simulink subsystem "PvtSubSys_PLAN_AP"  (R2020b)
settings: Solver=VariableStepAuto  StartTime=0.0  StopTime=10.0  RelTol=1e-3
undefined symbols (not defined in the file or in its folder): C_LongCtrl_0_Single, C_LongCtrl_0_Uint8, C_LongCtrl_Mph2Kph, magnitude, P_LongCtrl_accelTargAbsThrd, P_LongCtrl_AddVelAccelChange, P_LongCtrl_AddVelAccelThrd, P_LongCtrl_AddVelDistDesThrd, P_LongCtrl_AddVelEnable, P_LongCtrl_AddVelRefMsThrd, P_LongCtrl_ALaLowerChar, P_LongCtrl_ALaUpperCharEco, P_LongCtrl_ALaUpperCharNormal, P_LongCtrl_ALaUpperCharSport, P_LongCtrl_ALCAccLimitByDangerXAxis, P_LongCtrl_ALCAccLimitByDangerYAxis, P_LongCtrl_ALvAcceleLowerChar, P_LongCtrl_ALvAcceleUpperCharEco, P_LongCtrl_ALvAcceleUpperCharNormal, P_LongCtrl_ALvAcceleUpperCharSport, P_LongCtrl_CCaccelCCNeg2PosJerk, P_LongCtrl_CCaccelCCPosJerk, P_LongCtrl_CCaccelLowerIsLaneChange, P_LongCtrl_CCaccelMaxLCActive, P_LongCtrl_CCaccelMinECOAL, P_LongCtrl_CCaccelMinFastDecel, P_LongCtrl_CCaccelMinNoFastDecel, P_LongCtrl_CCaccelMinNormAL, P_LongCtrl_CCaccelMinSportAL, P_LongCtrl_CCaccelUpperCC, P_LongCtrl_CCaccelUpperCCSafeStop, P_LongCtrl_CCaMinNegAcceleLowerBand, P_LongCtrl_CCaMinNegAcceleUpperBand, P_LongCtrl_CCaMinPosAcceleLowerBand, P_LongCtrl_CCaMinPosAcceleUpperBand, P_LongCtrl_CCbECO, P_LongCtrl_CCbNorm, P_LongCtrl_CCbSport, P_LongCtrl_CCcoefESPSpd2IPSpd1, P_LongCtrl_CCcoefESPSpd2IPSpd2, P_LongCtrl_CCdecelCCJerk, P_LongCtrl_CCdecelCCJerkNegVLCInternalAcc, P_LongCtrl_CCfacNegAcceleLowerBand, P_LongCtrl_CCfacNegAcceleUpperBand, P_LongCtrl_CCfacPosAcceleLowerBand, P_LongCtrl_CCfacPosAcceleUpperBand, P_LongCtrl_CCkECO, P_LongCtrl_CCkNorm, P_LongCtrl_CCkSport, P_LongCtrl_CCLCIncSetSpdAdd, P_LongCtrl_CCLCIncSetSpdAddCntStartValue, P_LongCtrl_CCResumeDelayDeltaVel, P_LongCtrl_CCtAcceleTimeNeg, P_LongCtrl_CCtAcceleTimeNegCorrXAxis, P_LongCtrl_CCtAcceleTimeNegCorrYAxis, P_LongCtrl_CCtAcceleTimePos, P_LongCtrl_CCtAcceleTimePosCorrXAxis, P_LongCtrl_CCtAcceleTimePosCorrYAxis, P_LongCtrl_CCtStepVelPlan, P_LongCtrl_CCtTotVelPlan ... (+150)
libraries: simulink x62, TrueDurationTime x1
(part 1 of 7)
settings Model: Creator=GW00202955  LastModifiedBy=GW00235400

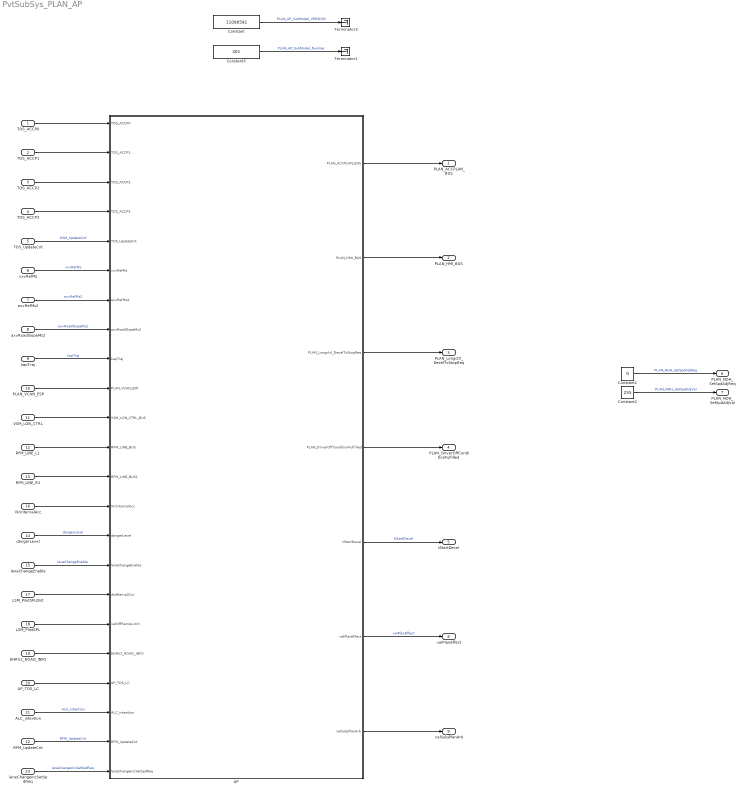
== system PvtSubSys_PLAN_AP ==
  TOS_ACCP0 : Inport  Description=|  OutDataTypeStr=Bus: TOS_ACCP0_BUS  PortDimensions=1  BusOutputAsStruct=on
      | IDP0     P0目标ID，确定目标是否切换
      | vxRelP0         P0目标相对速度，计算跟车加速度
      | axAbsGroundP0   P0目标绝对加速度，计算跟车加速度
      | rangeP0         P0目标相对距离，计算跟车加速度及P0动态距离
      | targetExistP0   P0目标是否存在，计算跟车加速度
      | ObjTypeP0       P0类型
  TOS_ACCP1 : Inport  Port=2  OutDataTypeStr=Bus: TOS_ACCP1_BUS  PortDimensions=1  BusOutputAsStruct=on
  TOS_ACCP2 : Inport  Description=|  Port=3  OutDataTypeStr=Bus: TOS_ACCP2_BUS  PortDimensions=1  BusOutputAsStruct=on
      | IDP2                 P2目标ID，确定目标是否切换
      | axAbsGroundP2        P2目标绝对加速度，计算P0目标绝对加速度滤波
      | rangeP2              P2目标相对距离，计算P2目标动态距离
      | targetExistP2        P2目标是否存在，计算P2目标动态距离
  TOS_ACCP3 : Inport  Description=|  Port=4  OutDataTypeStr=Bus: TOS_ACCP3_BUS  PortDimensions=1  BusOutputAsStruct=on
      | IDP3                 P3目标ID，确定目标是否切换
      | axAbsGroundP3        P3目标绝对加速度，计算P0目标绝对加速度滤波
      | rangeP3              P3目标相对距离，计算P2目标动态距离
      | targetExistP3        P3目标是否存在，计算P2目标动态距离
  TOS_UpdateCnt : Inport  Description=|目标是否更新  Port=5  OutDataTypeStr=uint32  PortDimensions=1  BusOutputAsStruct=on
  vxvRefMs : Inport  Description=m/s |车速  Port=6  OutDataTypeStr=single  PortDimensions=1  BusOutputAsStruct=on
  axvRefMs2 : Inport  Description=m/s^2 |自车参考加速度（未考虑CAN）  Port=7  OutDataTypeStr=single  PortDimensions=1  BusOutputAsStruct=on
  axvRoadSlopeMs2 : Inport  Description="m/s^2  |坡道加速度"  Port=8  OutDataTypeStr=single  PortDimensions=1  BusOutputAsStruct=on
  kapTraj : Inport  Description=1/m |方向盘转角计算弯道曲率，计算弯道工况加速度  Port=9  OutDataTypeStr=single  PortDimensions=1  BusOutputAsStruct=on
  PLAN_VCAN_ESP : Inport  Description=|  Port=10  OutDataTypeStr=Bus: VCAN_ESP_MSG_BUS  PortDimensions=1  BusOutputAsStruct=on
      | VehSpd   车速，用于计算仪表显示车速
      | DrivingModDis   驾驶模式
  VSM_LON_CTRL : Inport  Description=|  Port=11  OutDataTypeStr=Bus: VSM_LON_CTRL_BUS  PortDimensions=1  BusOutputAsStruct=on
      | ACCSts                 ACC状态
      | ACC_SpdSetValueKmh     驾驶员设定巡航速度
      | ACC_TimeGapSet         驾驶员设定车间时距
      | vSetBelowMin           驾驶员期望设定速度低于最小设定速度
      | HWAAccControlSts       HWA状态，用来判断换道进行中、safestop、HWA慢退
  RFM_LINE_L1 : Inport  Description=|  Port=12  OutDataTypeStr=Bus: RFM_LINE_BUS  PortDimensions=1  BusOutputAsStruct=on
      | dC0V          左侧车道线三次多项式常数项系数
      | dC1V          左侧车道线三次多项式一次项系数     
      | dC2V          左侧车道线三次多项式二次项系数  
      | dC3V          左侧车道线三次多项式三次项系数  
      | dDisFront     车辆坐标系X方向车道线置信距离
      | bIsLineExist  车道线存在
  RFM_LINE_R1 : Inport  Description=|  Port=13  OutDataTypeStr=Bus: RFM_LINE_BUS  PortDimensions=1  BusOutputAsStruct=on
      | dC0V          右侧车道线三次多项式常数项系数
      | dC1V          右侧车道线三次多项式一次项系数     
      | dC2V          右侧车道线三次多项式二次项系数  
      | dC3V          右侧车道线三次多项式三次项系数  
      | dDisFront     车辆坐标系X方向车道线置信距离
      | bIsLineExist  车道线存在
  dangerLevel : Inport  Description=|换道危险程度，抑制换道减速度  Port=14  OutDataTypeStr=single  PortDimensions=1
  laneChangeEnable : Inport  Description=|换道条件满足，用作换道减速度抑制开启条件  Port=15  OutDataTypeStr=boolean  PortDimensions=1
  VlcInternalAcc : Inport  Description=m/s^2 |VLC执行加速度，用作当前加速度判断  Port=16  OutDataTypeStr=single  PortDimensions=1
  LSM_PilotSPLDist : Inport  Description=m |到匝道距离  Port=17  OutDataTypeStr=uint16  PortDimensions=1
  LSM_PilotSPL : Inport  Description=km/h |匝道限速  Port=18  OutDataTypeStr=uint8  PortDimensions=1
  EHRV2_ROAD_INFO : Inport  Description=|  Port=19  OutDataTypeStr=Bus: EHRV2_ROAD_INFO_BUS
      | i_road_curvature                    当前车辆位置处曲率(左正右负)
      | i_road_curvature_far                当前车辆位置前方Xm内最大曲率(左正右负)
      | i_road_curvature_far_distance       当前车辆位置与前方Xm内最大曲率点相对距离
      | i_road_curvature_value_matrix       车辆所在车道道路记录点的曲率组成的矩阵
      | i_road_curvature_distance_matrix    车辆坐标系下道路记录点的x坐标组成的矩阵
      | i_road_curvature_matrix_size        车辆所在车道道路记录点的个数
  AP_TOS_LC : Inport  Description=|  Port=20  OutDataTypeStr=Bus: TOS_LC_BUS
      | Object_ID             融合追踪处理后，目标的ID
      | Object_Type           目标的类型（行人、小汽车、卡车...）
      | Object_Length         目标的长度
      | Object_Width          目标的宽度
      | Object_Hight          目标的高度
      | Object_DX             车体坐标系下，自车和目标纵向相对距离
      | Object_DY             车体坐标系下，自车和目标横向相对距离
      | Object_VX             目标的纵向的速度
      | Object_VY             目标的横向的速度
      | Object_HeadingAngle   车体系下, 目标航向角
      | Object_Fus_Type       目标是否是融合,传感器类型
      | Object_ExistProb      目标存在的可能性
      | Object_ObstacleProb   目标成为障碍物的概率值
      | Object_Age            目标存在生命周期
      | Object_AX             目标的纵向的加速度
  ALC_intention : Inport  Description="|  换到意图 -1右换道，0不换"  Port=21  OutDataTypeStr=int8  PortDimensions=1
  RFM_UpdateCnt : Inport  Description=|RFM更新周期  Port=22  OutDataTypeStr=uint32  PortDimensions=1
  laneChangeIncSetSpdReq : Inport  Description=|换道加速开启条件  Port=23  OutDataTypeStr=uint8  PortDimensions=1
  AP : Subsystem  Description=Acceleration Plan
  Constant : Constant  Value=11090591  OutDataTypeStr=uint32
  Constant1 : Constant  Value=0  OutDataTypeStr=boolean
  Constant2 : Constant  Value=255  OutDataTypeStr=uint8
  Constant3 : Constant  Value=301  OutDataTypeStr=uint32
  Terminator1 : Terminator
  Terminator3 : Terminator
  PLAN_ACCPLAN_BUS : Outport  Description=|  OutDataTypeStr=Bus: PLAN_ACCPLAN_BUS
      | ACC_axvCvAim                      期望加速度
      | ACC_axv_ComfortBandLowerValue     期望加速度下限
      | ACC_axv_ComfortBandUpperValue     期望加速度上限
      | ACC_DecelerateJerk                加速度变化率下限
      | ACC_AccelerateJerk                加速度变化率上限         
      | ACC_BrakePrefer                   制动优先
  PLAN_HMI_BUS : Outport  Description=|  Port=2  OutDataTypeStr=Bus: PLAN_HMI_BUS
      | tor                       驾驶员接管请求
      | ACC_TgtObjBarDisp         P0动态距离
      | ACC_LeTgtObjBarDisp       P2动态距离
      | ACC_RiTgtObjBarDisp       P3动态距离
      | IntelligentCurveActive    智能过弯激活状态
  PLAN_Longctrl_DecelToStopReq : Outport  Description=|制动到停状态  Port=3  OutDataTypeStr=boolean  PortDimensions=1
  PLAN_DriverOffConditionFulfilled : Outport  Description=|起步条件满足  Port=4  OutDataTypeStr=boolean  PortDimensions=1
  tStartDecel : Outport  Port=5
  PLAN_NOH_SetSpdAdjReq : Outport  Port=6  OutDataTypeStr=boolean
  PLAN_NOH_SetSpdAdjVal : Outport  Port=7  OutDataTypeStr=uint8
  velPlanEffect : Outport  Port=8
  velSubjPlanArb : Outport  Port=9
  wires:
  VSM_LON_CTRL/1 -> AP/11(VSM_LON_CTRL_BUS)
  Constant3/1 -> Terminator1/1  "PLAN_AP_SubModel_Number"
  laneChangeIncSetSpdReq/1 -> AP/23(laneChangeIncSetSpdReq)  "laneChangeIncSetSpdReq"
  axvRoadSlopeMs2/1 -> AP/8(axvRoadSlopeMs2)  "axvRoadSlopeMs2"
  LSM_PilotSPL/1 -> AP/18(velOffRampLimit)
  dangerLevel/1 -> AP/15(dangerLevel)  "dangerLevel"
  AP/2(PLAN_HMI_BUS) -> PLAN_HMI_BUS/1
  TOS_UpdateCnt/1 -> AP/5(TOS_UpdateCnt)  "OSM_UpdateCnt"
  LSM_PilotSPLDist/1 -> AP/17(distRamp2Cur)
  AP/1(PLAN_ACCPLAN_BUS) -> PLAN_ACCPLAN_BUS/1
  Constant/1 -> Terminator3/1  "PLAN_AP_SubModel_VERSION"
  vxvRefMs/1 -> AP/6(vxvRefMs)  "vxvRefMs"
  kapTraj/1 -> AP/9(kapTraj)  "kapTraj"
  TOS_ACCP1/1 -> AP/2(TOS_ACCP1)
  RFM_LINE_R1/1 -> AP/13(RFM_LINE_BUS1)
  TOS_ACCP2/1 -> AP/3(TOS_ACCP2)
  TOS_ACCP0/1 -> AP/1(TOS_ACCP0)
  AP/3(PLAN_Longctrl_DecelToStopReq) -> PLAN_Longctrl_DecelToStopReq/1
  PLAN_VCAN_ESP/1 -> AP/10(PLAN_VCAN_ESP)
  AP/5(tStartDecel) -> tStartDecel/1  "tStartDecel"
  Constant1/1 -> PLAN_NOH_SetSpdAdjReq/1  "PLAN_NOH_SetSpdAdjReq"
  RFM_UpdateCnt/1 -> AP/22(RFM_UpdateCnt)  "RFM_UpdateCnt"
  TOS_ACCP3/1 -> AP/4(TOS_ACCP3)
  VlcInternalAcc/1 -> AP/14(VlcInternalAcc)
  ALC_intention/1 -> AP/21(ALC_intention)  "ALC_intention"
  RFM_LINE_L1/1 -> AP/12(RFM_LINE_BUS)
  Constant2/1 -> PLAN_NOH_SetSpdAdjVal/1  "PLAN_NOH_SetSpdAdjVal"
  laneChangeEnable/1 -> AP/16(laneChangeEnable)  "laneChangeEnable"
  axvRefMs2/1 -> AP/7(axvRefMs2)  "axvRefMs2"
  AP/7(velSubjPlanArb) -> velSubjPlanArb/1
  AP/4(PLAN_DriverOffConditionFulfilled) -> PLAN_DriverOffConditionFulfilled/1
  EHRV2_ROAD_INFO/1 -> AP/19(EHRV2_ROAD_INFO)
  AP/6(velPlanEffect) -> velPlanEffect/1  "velPlanEffect"
  AP_TOS_LC/1 -> AP/20(AP_TOS_LC)

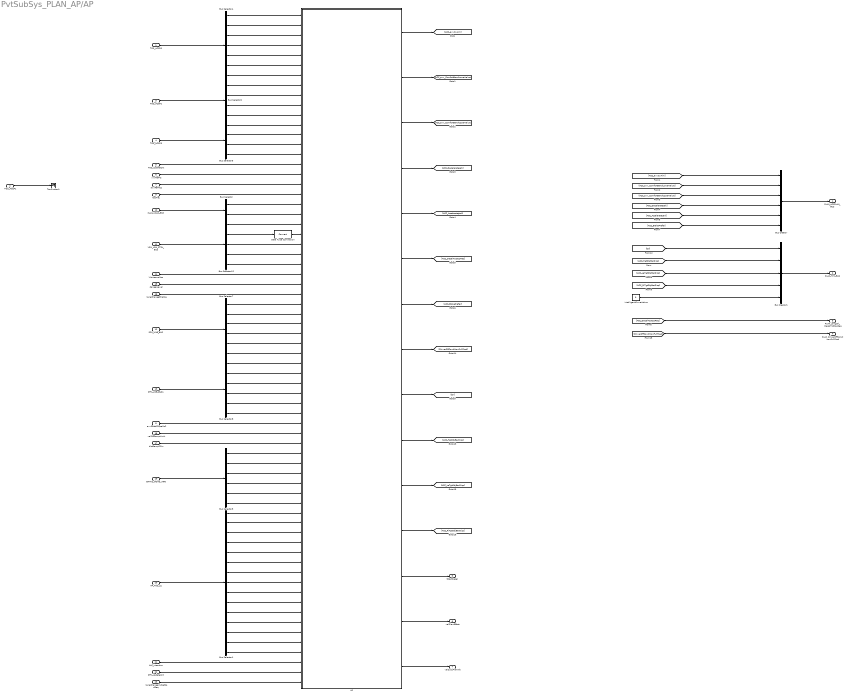
== system PvtSubSys_PLAN_AP/AP ==
  TOS_ACCP0 : Inport  OutDataTypeStr=Bus: TOS_ACCP0_BUS  LockScale=on
  TOS_ACCP1 : Inport  Port=2  OutDataTypeStr=Bus: TOS_ACCP1_BUS
  TOS_ACCP2 : Inport  Port=3  OutDataTypeStr=Bus: TOS_ACCP2_BUS
  TOS_ACCP3 : Inport  Port=4  OutDataTypeStr=Bus: TOS_ACCP3_BUS
  TOS_UpdateCnt : Inport  Port=5
  vxvRefMs : Inport  Port=6
  axvRefMs2 : Inport  Port=7
  axvRoadSlopeMs2 : Inport  Port=8
  kapTraj : Inport  Port=9
  PLAN_VCAN_ESP : Inport  Port=10  OutDataTypeStr=Bus: VCAN_ESP_MSG_BUS
  VSM_LON_CTRL_BUS : Inport  Port=11  OutDataTypeStr=Bus: VSM_LON_CTRL_BUS
  RFM_LINE_BUS : Inport  Port=12  OutDataTypeStr=Bus: RFM_LINE_BUS
  RFM_LINE_BUS1 : Inport  Port=13  OutDataTypeStr=Bus: RFM_LINE_BUS
  VlcInternalAcc : Inport  Port=14
  dangerLevel : Inport  Port=15
  laneChangeEnable : Inport  Port=16
  distRamp2Cur : Inport  Port=17  OutDataTypeStr=uint16
  velOffRampLimit : Inport  Port=18  OutDataTypeStr=uint8
  EHRV2_ROAD_INFO : Inport  Port=19  OutDataTypeStr=Bus: EHRV2_ROAD_INFO_BUS
  AP_TOS_LC : Inport  Port=20  OutDataTypeStr=Bus: TOS_LC_BUS
  ALC_intention : Inport  Port=21
  RFM_UpdateCnt : Inport  Port=22  OutDataTypeStr=uint32
  laneChangeIncSetSpdReq : Inport  Port=23  OutDataTypeStr=uint8
  AP : Subsystem  Description=Acceleration Plan  TreatAsAtomicUnit=on
  Bus Creator : BusCreator  Inputs=6  OutDataTypeStr=Bus: PLAN_ACCPLAN_BUS  NonVirtualBus=on
      settings: InheritFromInputs=off
  Bus Creator1 : BusCreator  Inputs=5  OutDataTypeStr=Bus: PLAN_HMI_BUS  NonVirtualBus=on
      settings: InheritFromInputs=off
  Bus Selector : BusSelector  OutputSignals=VehSpd,DrivingModDis
  Bus Selector1 : BusSelector  OutputSignals=Object_ID,Object_Type,Object_Length,Object_Width,Object_Hight,Object_DX,Object_DY,Object_VX,Object_VY,Object_HeadingAngle,Object_Fus_Type,Object_ExistProb,Object_ObstacleProb,Object_Age,Object_AX
  Bus Selector12 : BusSelector  OutputSignals=ACCSts,ACC_SpdSetValueKmh,ACC_TimeGapSet,vSetBelowMin,HWAAccControlSts
  Bus Selector2 : BusSelector  OutputSignals=IDP2,axAbsGroundP2,rangeP2,targetExistP2
  Bus Selector3 : BusSelector  OutputSignals=i_road_curvature,i_road_curvature_far,i_road_curvature_far_distance,i_road_curvature_value_matrix,i_road_curvature_distance_matrix,i_road_curvature_matrix_size
  Bus Selector4 : BusSelector  OutputSignals=IDP0,vxRelP0,axAbsGroundP0,rangeP0,targetExistP0,ObjTypeP0,ObjMovingStateP0
  Bus Selector5 : BusSelector  OutputSignals=IDP3,axAbsGroundP3,rangeP3,targetExistP3
  Bus Selector7 : BusSelector  OutputSignals=dC0V,dC1V,dC2V,dC3V,dDisFront,bIsLineExist
  Bus Selector8 : BusSelector  OutputSignals=dC0V,dC1V,dC2V,dC3V,dDisFront,bIsLineExist
  Data Type Conversion : DataTypeConversion
  IntelligentCurveActive : Constant  Value=0  OutDataTypeStr=boolean
  Terminator1 : Terminator
  PLAN_ACCPLAN_BUS : Outport  OutDataTypeStr=Bus: PLAN_ACCPLAN_BUS
  PLAN_HMI_BUS : Outport  Port=2  OutDataTypeStr=Bus: PLAN_HMI_BUS
  PLAN_Longctrl_DecelToStopReq : Outport  Port=3  OutDataTypeStr=boolean
  PLAN_DriverOffConditionFulfilled : Outport  Port=4  OutDataTypeStr=boolean
  tStartDecel : Outport  Port=5  OutDataTypeStr=single
  velPlanEffect : Outport  Port=6  OutDataTypeStr=uint8
  velSubjPlanArb : Outport  Port=7  OutDataTypeStr=single
  wires:
  Bus Selector4/7 -> AP/7(ObjMovingStateP0)  "<ObjMovingStateP0>"
  Bus Selector4/6 -> AP/6(ObjTypeP0)  "<ObjTypeP0>"
  RFM_UpdateCnt/1 -> AP/67(RFM_UpdateCnt)  "RFM_UpdateCnt"
  Bus Selector1/4 -> AP/54(Object_Width)  "<Object_Width>"
  Bus Selector1/9 -> AP/59(Object_VY)  "<Object_VY>"
  Bus Selector1/11 -> AP/61(Object_Fus_Type)  "<Object_Fus_Type>"
  Bus Selector1/8 -> AP/58(Object_VX)  "<Object_VX>"
  Bus Selector3/4 -> AP/48(i_road_curvature_value_matrix)  "<i_road_curvature_value_matrix>"
  Bus Selector1/13 -> AP/63(Object_ObstacleProb)  "<Object_ObstacleProb>"
  Bus Selector1/12 -> AP/62(Object_ExistProb)  "<Object_ExistProb>"
  Bus Selector1/15 -> AP/65(Object_AX)  "<Object_AX>"
  Bus Selector1/14 -> AP/64(Object_Age)  "<Object_Age>"
  Bus Selector3/1 -> AP/45(i_road_curvature)  "<i_road_curvature>"
  Bus Selector3/5 -> AP/49(i_road_curvature_distance_matrix)  "<i_road_curvature_distance_matrix>"
  Bus Selector1/5 -> AP/55(Object_Hight)  "<Object_Hight>"
  Bus Selector1/3 -> AP/53(Object_Length)  "<Object_Length>"
  EHRV2_ROAD_INFO/1 -> Bus Selector3/1
  Bus Selector1/1 -> AP/51(Object_ID)  "<Object_ID>"
  AP_TOS_LC/1 -> Bus Selector1/1
  Bus Selector1/2 -> AP/52(Object_Type)  "<Object_Type>"
  Bus Selector1/10 -> AP/60(Object_HeadingAngle)  "<Object_HeadingAngle>"
  Bus Selector1/6 -> AP/56(Object_DX)  "<Object_DX>"
  Bus Selector3/2 -> AP/46(i_road_curvature_far)  "<i_road_curvature_far>"
  Bus Selector1/7 -> AP/57(Object_DY)  "<Object_DY>"
  ALC_intention/1 -> AP/66(ALC_intention)  "ALC_intention"
  Bus Selector3/3 -> AP/47(i_road_curvature_far_distance)  "<i_road_curvature_far_distance>"
  Bus Selector3/6 -> AP/50(i_road_curvature_matrix_size)  "<i_road_curvature_matrix_size>"
  Bus Selector8/2 -> AP/37(R1dC1V)  "<dC1V>"
  Bus Selector8/1 -> AP/36(R1dC0V)  "<dC0V>"
  Bus Selector7/6 -> AP/35(L1bIsLineExist)  "<bIsLineExist>"
  Bus Selector7/5 -> AP/34(L1dDisFront)  "<dDisFront>"
  Bus Selector7/4 -> AP/33(L1dC3V)  "<dC3V>"
  Bus Selector7/3 -> AP/32(L1dC2V)  "<dC2V>"
  Bus Selector7/2 -> AP/31(L1dC1V)  "<dC1V>"
  Bus Selector7/1 -> AP/30(L1dC0V)  "<dC0V>"
  [ACC_RiTgtObjBarDisp] -> Bus Creator1/4  "ACC_RiTgtObjBarDisp"
  [ACC_LeTgtObjBarDisp] -> Bus Creator1/3  "ACC_LeTgtObjBarDisp"
  [ACC_TgtObjBarDisp] -> Bus Creator1/2  "ACC_TgtObjBarDisp"
  Bus Creator/1 -> PLAN_ACCPLAN_BUS/1
  Bus Selector8/6 -> AP/41(R1bIsLineExis)  "<bIsLineExist>"
  Bus Selector8/5 -> AP/40(R1dDisFront)  "<dDisFront>"
  Bus Selector8/4 -> AP/39(R1dC3V)  "<dC3V>"
  Bus Selector8/3 -> AP/38(R1dC2V)  "<dC2V>"
  AP/13(tStartDecel) -> tStartDecel/1  "tStartDecel"
  laneChangeEnable/1 -> AP/29(laneChangeEnable)  "laneChangeEnable"
  dangerLevel/1 -> AP/28(dangerLevel)  "dangerLevel"
  Bus Selector12/5 -> AP/26(HWAAccControlSts)  "<HWAAccControlSts>"
  Bus Selector12/4 -> AP/25(vSetBelowMin)  "<vSetBelowMin>"
  Bus Selector5/2 -> AP/13(accelTargAbsP3)  "<axAbsGroundP3>"
  Bus Selector5/1 -> AP/12(IDP3)  "<IDP3>"
  Bus Selector2/2 -> AP/9(accelTargAbsP2)  "<axAbsGroundP2>"
  Bus Selector2/1 -> AP/8(IDP2)  "<IDP2>"
  Data Type Conversion/1 -> AP/23(ACC_SpdSetValue)
  RFM_LINE_BUS1/1 -> Bus Selector8/1
  RFM_LINE_BUS/1 -> Bus Selector7/1
  kapTraj/1 -> AP/19(kap)  "kapTraj"
  axvRoadSlopeMs2/1 -> AP/42(axvRoadSlopeMs2)  "axvRoadSlopeMs2"
  TOS_ACCP3/1 -> Bus Selector5/1
  TOS_ACCP2/1 -> Bus Selector2/1
  TOS_ACCP1/1 -> Terminator1/1
  Bus Selector12/3 -> AP/24(timeGap)  "<ACC_TimeGapSet>"
  Bus Selector12/2 -> Data Type Conversion/1  "<ACC_SpdSetValueKmh>"
  Bus Selector12/1 -> AP/22(ACCModeSts)  "<ACCSts>"
  Bus Selector4/5 -> AP/5(targetExistP0)  "<targetExistP0>"
  Bus Selector4/4 -> AP/4(distTargRel)  "<rangeP0>"
  Bus Selector4/3 -> AP/3(accelTargAbsP0)  "<axAbsGroundP0>"
  Bus Selector4/2 -> AP/2(velTargRel)  "<vxRelP0>"
  Bus Selector4/1 -> AP/1(IDP0)  "<IDP0>"
  AP/12(ACC_RiTgtObjBarDisp) -> [ACC_RiTgtObjBarDisp]
  AP/11(ACC_LeTgtObjBarDisp) -> [ACC_LeTgtObjBarDisp]
  AP/10(ACC_TgtObjBarDisp) -> [ACC_TgtObjBarDisp]  "ACC_TgtObjBarDisp"
  AP/9(tor) -> [tor]
  AP/8(DriveOffConditonFulfilled) -> [DriverOffConditionFulfilled]  "DriverOffConditionFulfilled"
  AP/7(BrakePrefer) -> [ACC_BrakePrefer]  "ACC_BrakePrefer"
  AP/6(DecleToStop) -> [ACC_DecelToStopReq]  "ACC_DecelToStopReq"
  AP/5(upperJerkAL) -> [ACC_AccelerateJerk]  "ACC_AccelerateJerk"
  AP/4(lowerJerkAL) -> [ACC_DecelerateJerk]  "ACC_DecelerateJerk"
  AP/3(upperBandAL) -> [ACC_axv_ComfortBandUpperValue]  "ACC_axv_ComfortBandUpperValue"
  AP/2(lowerBandAL) -> [ACC_axv_ComfortBandLowerValue]  "ACC_axv_ComfortBandLowerValue"
  AP/1(accelAL) -> [ACC_axvCvAim]  "ACC_axvCvAim"
  [ACC_axv_ComfortBandUpperValue] -> Bus Creator/3  "ACC_axv_ComfortBandUpperValue"
  VSM_LON_CTRL_BUS/1 -> Bus Selector12/1
  PLAN_VCAN_ESP/1 -> Bus Selector/1
  Bus Selector/2 -> AP/21(DrivingMode)  "<DrivingModDis>"
  Bus Selector/1 -> AP/20(VehicleSpd)  "<VehSpd>"
  axvRefMs2/1 -> AP/18(accelSubj)  "axvRefMs2"
  vxvRefMs/1 -> AP/17(velSubj)  "vxvRefMs"
  TOS_ACCP0/1 -> Bus Selector4/1
  [DriverOffConditionFulfilled] -> PLAN_DriverOffConditionFulfilled/1  "PLAN_DriverOffConditionFulfilled"
  TOS_UpdateCnt/1 -> AP/16(TOS_UpdateCnt)  "OSM_UpdateCnt"
  [ACC_AccelerateJerk] -> Bus Creator/5  "ACC_AccelerateJerk"
  [ACC_DecelerateJerk] -> Bus Creator/4  "ACC_DecelerateJerk"
  VlcInternalAcc/1 -> AP/27(VlcInternalAccK1)  "VlcInternalAcc"
  [ACC_axv_ComfortBandLowerValue] -> Bus Creator/2  "ACC_axv_ComfortBandLowerValue"
  [ACC_DecelToStopReq] -> PLAN_Longctrl_DecelToStopReq/1  "PLAN_Longctrl_DecelToStopReq"
  [ACC_axvCvAim] -> Bus Creator/1  "ACC_axvCvAim"
  [ACC_BrakePrefer] -> Bus Creator/6  "ACC_BrakePrefer"
  [tor] -> Bus Creator1/1  "tor"
  IntelligentCurveActive/1 -> Bus Creator1/5  "IntelligentCurveActive"
  Bus Creator1/1 -> PLAN_HMI_BUS/1
  Bus Selector2/3 -> AP/10(distTargRelP2)  "<rangeP2>"
  Bus Selector2/4 -> AP/11(P2_Exist)  "<targetExistP2>"
  Bus Selector5/3 -> AP/14(distTargRelP3)  "<rangeP3>"
  Bus Selector5/4 -> AP/15(P3_Exist)  "<targetExistP3>"
  velOffRampLimit/1 -> AP/43(velOffRampLimit)  "velOffRampLimit"
  distRamp2Cur/1 -> AP/44(distRamp2Cur)  "distRamp2Cur"
  AP/14(velPlanEffect) -> velPlanEffect/1  "velPlanEffect"
  AP/15(velSubjPlanArb) -> velSubjPlanArb/1
  laneChangeIncSetSpdReq/1 -> AP/68(laneChangeIncSetSpdReq)  "laneChangeIncSetSpdReq"

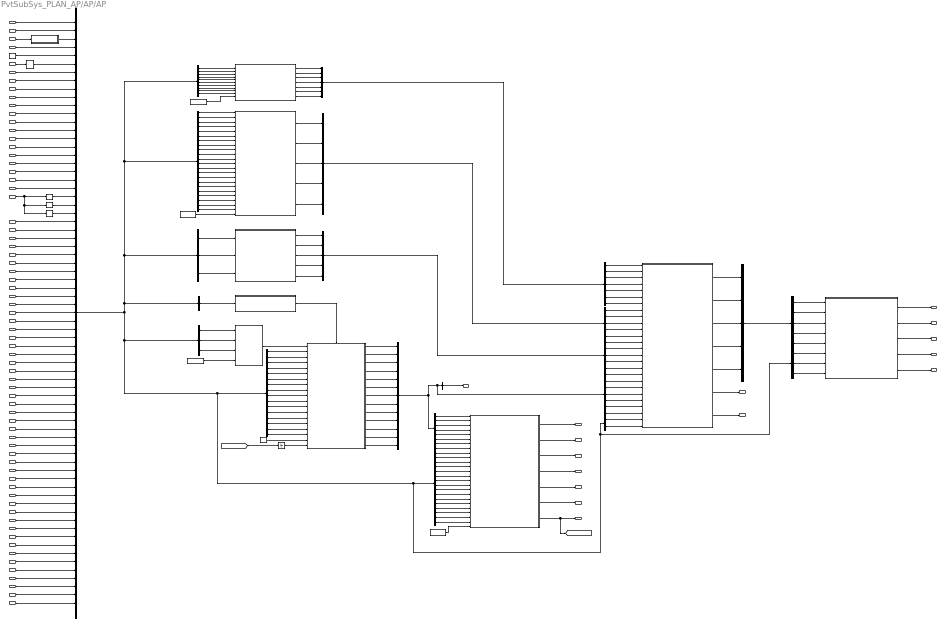
== system PvtSubSys_PLAN_AP/AP/AP ==
  note: Note:
  note: If Follow moudle's runtime is changed,should be changed together as followed:tCycle and jerk in decelToStop moudle.
  IDP0 : Inport  OutDataTypeStr=uint8
  velTargRel : Inport  Port=2  OutDataTypeStr=single  Interpolate=off
  accelTargAbsP0 : Inport  Port=3  OutDataTypeStr=single  Interpolate=off
  distTargRel : Inport  Port=4  OutDataTypeStr=single  Interpolate=off
  targetExistP0 : Inport  Port=5  OutDataTypeStr=boolean  Interpolate=off
  ObjTypeP0 : Inport  Port=6
  ObjMovingStateP0 : Inport  Port=7
  IDP2 : Inport  Port=8  OutDataTypeStr=uint8
  accelTargAbsP2 : Inport  Port=9  OutDataTypeStr=single
  distTargRelP2 : Inport  Port=10
  P2_Exist : Inport  Port=11
  IDP3 : Inport  Port=12  OutDataTypeStr=uint8
  accelTargAbsP3 : Inport  Port=13  OutDataTypeStr=single
  distTargRelP3 : Inport  Port=14
  P3_Exist : Inport  Port=15
  TOS_UpdateCnt : Inport  Port=16  OutDataTypeStr=uint32
  velSubj : Inport  Port=17  OutDataTypeStr=single  Interpolate=off
  accelSubj : Inport  Port=18  OutDataTypeStr=single  Interpolate=off
  kap : Inport  Port=19  OutDataTypeStr=single
  VehicleSpd : Inport  Port=20  OutDataTypeStr=single  Interpolate=off
  DrivingMode : Inport  Port=21  OutDataTypeStr=uint8
  ACCModeSts : Inport  Port=22  OutDataTypeStr=uint8  Interpolate=off
  ACC_SpdSetValue : Inport  Port=23  OutDataTypeStr=single  Interpolate=off
  timeGap : Inport  Port=24  OutDataTypeStr=uint8  Interpolate=off
  vSetBelowMin : Inport  Port=25  OutDataTypeStr=boolean
  HWAAccControlSts : Inport  Port=26  OutDataTypeStr=uint8
  VlcInternalAccK1 : Inport  Port=27  OutDataTypeStr=single  Interpolate=off
  dangerLevel : Inport  Port=28  OutDataTypeStr=single
  laneChangeEnable : Inport  Port=29  OutDataTypeStr=boolean
  L1dC0V : Inport  Port=30  OutDataTypeStr=single
  L1dC1V : Inport  Port=31  OutDataTypeStr=single
  L1dC2V : Inport  Port=32  OutDataTypeStr=single
  L1dC3V : Inport  Port=33  OutDataTypeStr=single
  L1dDisFront : Inport  Port=34  OutDataTypeStr=single
  L1bIsLineExist : Inport  Port=35
  R1dC0V : Inport  Port=36  OutDataTypeStr=single
  R1dC1V : Inport  Port=37  OutDataTypeStr=single
  R1dC2V : Inport  Port=38  OutDataTypeStr=single
  R1dC3V : Inport  Port=39  OutDataTypeStr=single
  R1dDisFront : Inport  Port=40  OutDataTypeStr=single
  R1bIsLineExis : Inport  Port=41
  axvRoadSlopeMs2 : Inport  Port=42
  velOffRampLimit : Inport  Port=43
  distRamp2Cur : Inport  Port=44
  i_road_curvature : Inport  Port=45
  i_road_curvature_far : Inport  Port=46
  i_road_curvature_far_distance : Inport  Port=47
  i_road_curvature_value_matrix : Inport  Port=48
  i_road_curvature_distance_matrix : Inport  Port=49
  i_road_curvature_matrix_size : Inport  Port=50
  Object_ID : Inport  Port=51
  Object_Type : Inport  Port=52
  Object_Length : Inport  Port=53
  Object_Width : Inport  Port=54
  Object_Hight : Inport  Port=55
  Object_DX : Inport  Port=56
  Object_DY : Inport  Port=57
  Object_VX : Inport  Port=58
  Object_VY : Inport  Port=59
  Object_HeadingAngle : Inport  Port=60
  Object_Fus_Type : Inport  Port=61
  Object_ExistProb : Inport  Port=62
  Object_ObstacleProb : Inport  Port=63
  Object_Age : Inport  Port=64
  Object_AX : Inport  Port=65
  ALC_intention : Inport  Port=66
  RFM_UpdateCnt : Inport  Port=67  OutDataTypeStr=uint32
  laneChangeIncSetSpdReq : Inport  Port=68  OutDataTypeStr=uint8
  AL : Subsystem  Description=Acceleration Limition
  Arbitrate : Subsystem
  Bus Creator : BusCreator  Inputs=7
  Bus Creator1 : BusCreator  Inputs=13
  Bus Creator10 : BusCreator  Inputs=5
  Bus Creator2 : BusCreator  Inputs=5
  Bus Creator3 : BusCreator  Inputs=71
  Bus Creator5 : BusCreator  Inputs=5
  Bus Selector : BusSelector  OutputSignals=accelCC,upperBandCC,lowerBandCC,upperJerkCC,lowerJerkCC,accelCCCtrlAfterJerk,velSubjPlanCC2ALC
  Bus Selector1 : BusSelector  OutputSignals=accelFollow,accelFollowAfterJerk,upperBandFollow,lowerBandFollow,upperJerkFollow,lowerJerkFollow,velSubjPlanFollow
  Bus Selector10 : BusSelector  OutputSignals=LongCtrl_DrivingMode,velSubj,HWASlowQuit
  Bus Selector11 : BusSelector  OutputSignals=velSubj,kap,L1dC0V,L1dC1V,L1dC2V,L1dC3V,R1dC0V,R1dC1V,R1dC2V,R1dC3V,L1dDisFront,R1dDisFront,L1bIsLineExist,R1bIsLineExis,VlcInternalAccK1,i_road_curvature,i_road_curvature_far,i_road_curvature_far_distance,i_road_curvature_value_matrix,i_road_curvature_distance_matrix,i_road_curvature_matrix_size,RFM_UpdateCnt
  Bus Selector12 : BusSelector  OutputSignals=accelIC,upperBandIC,lowerBandIC,upperJerkIC,lowerJerkIC
  Bus Selector13 : BusSelector  OutputSignals=velOffRampLimit,distRamp2Cur,vehicleSpd
  Bus Selector14 : BusSelector  OutputSignals=accelORD,upperBandORD,lowerBandORD,upperJerkORD,lowerJerkORD
  Bus Selector15 : BusSelector  OutputSignals=tStartDecel
  Bus Selector2 : BusSelector  OutputSignals=accelArb,upperBandArb,lowerBandArb,upperJerkArb,lowerJerkArb
  Bus Selector3 : BusSelector  OutputSignals=accelFollow,distDesCur,distRelPlanMin,distRelDesDistRelPlanNumMin,ttc,accelSubjPlanOpt
  Bus Selector4 : BusSelector  OutputSignals=ACC_SpdSetValue,vehicleSpd,IP_VehSpdUnit,VlcInternalAccK1,vSetBelowMin,HWAIsLaneChange,SafeStopActive,LongCtrl_DrivingMode,velSubj,laneChangeIncSetSpdReq
  Bus Selector5 : BusSelector  OutputSignals=TOS_UpdateCnt
  Bus Selector6 : BusSelector  OutputSignals=VlcInternalAccK1,ACCModeSts,accelSubj
  Bus Selector7 : BusSelector  OutputSignals=velSubj,VlcInternalAccK1,distTargRel,velTargRel,accelTargAbsP0,timeGap,ACCModeSts,IDP0,IDP2,IDP3,accelTargAbsP2,accelTargAbsP3,dangerLevel,laneChangeEnable,axvRoadSlopeMs2,ObjMovingStateP0
  Bus Selector8 : BusSelector  OutputSignals=velSubj,targetExistP0,distTargRel,velTargRel,ACC_SpdSetValue,ACCModeSts,VlcInternalAccK1,timeGap,SafeStopActive,distTargRelP2,P2_Exist,distTargRelP3,P3_Exist,axvRoadSlopeMs2,accelSubj,VlcInternalAccK1,HWASlowQuit,ObjTypeP0
  Bus Selector9 : BusSelector  OutputSignals=targetExistP0,ACCModeSts
  CCCtrl : Subsystem  Description=Cruise Control
  Compare To Constant1 : simulink/Logic and Bit Operations/Compare To Constant  relop===  const=3  OutDataTypeStr=boolean
  Compare To Constant10 : simulink/Logic and Bit Operations/Compare To Constant  relop===  const=2  OutDataTypeStr=boolean
  Compare To Constant2 : simulink/Logic and Bit Operations/Compare To Constant  relop===  const=5  OutDataTypeStr=boolean
  Constant : Constant  Value=0  OutDataTypeStr=uint8
  FollowCtrl : Subsystem
  FollowtCycle : Constant  Value=0.05  OutDataTypeStr=single
  IC : Subsystem  Description=Intelligence Curve
  ORD : Subsystem  Description=Off Ramp Decelerate
  P_LongCtrltCycle{,1..2,6} (4 alike) : Constant  Value=P_LongCtrl_tCycle  OutDataTypeStr=single
  SJ : Subsystem  Description=State Judge
  Signal Copy : SignalConversion  OverrideOpt=off
  Subsystem : Subsystem
  TargetUpdate : Subsystem
  Unit Delay : UnitDelay  SampleTime=-1  HasFrameUpgradeWarning=on
  VlcInternalAccCalc : Subsystem
  accelAL : Outport  OutDataTypeStr=single
  lowerBandAL : Outport  Port=2  OutDataTypeStr=single
  upperBandAL : Outport  Port=3  OutDataTypeStr=single
  lowerJerkAL : Outport  Port=4  OutDataTypeStr=single
  upperJerkAL : Outport  Port=5  OutDataTypeStr=single
  DecleToStop : Outport  Port=6  OutDataTypeStr=boolean
  BrakePrefer : Outport  Port=7  OutDataTypeStr=boolean
  DriveOffConditonFulfilled : Outport  Port=8  OutDataTypeStr=boolean
  tor : Outport  Port=9  OutDataTypeStr=boolean
  ACC_TgtObjBarDisp : Outport  Port=10  OutDataTypeStr=uint8
  ACC_LeTgtObjBarDisp : Outport  Port=11  OutDataTypeStr=uint8
  ACC_RiTgtObjBarDisp : Outport  Port=12  OutDataTypeStr=uint8
  tStartDecel : Outport  Port=13  OutDataTypeStr=single
  velPlanEffect : Outport  Port=14  OutDataTypeStr=uint8
  velSubjPlanArb : Outport  Port=15  OutDataTypeStr=single
  wires:
  P_LongCtrltCycle2/1 -> SJ/25(tCycle)
  Signal Copy/1 -> Bus Creator3/6  "LongCtrl_DrivingMode"
  Bus Selector7/16 -> FollowCtrl/17(ObjMovingStateP0)  "<ObjMovingStateP0>"
  ObjMovingStateP0/1 -> Bus Creator3/71  "ObjMovingStateP0"
  Bus Selector8/18 -> SJ/24(ObjTypeP0)  "<ObjTypeP0>"
  ObjTypeP0/1 -> Bus Creator3/20  "ObjTypeP0"
  Bus Selector10/3 -> AL/8(HWASlowQuit)  "<HWASlowQuit>"
  ACCModeSts/1 -> Subsystem/1(u)  "ACCModeSts"
  Bus Selector11/17 -> IC/17(i_road_curvature_far)  "<i_road_curvature_far>"
  Bus Selector11/9 -> IC/9(R1dC2V)  "<R1dC2V>"
  IC/2(upperBandIC) -> Bus Creator10/2  "upperBandIC"
  Bus Selector11/18 -> IC/18(i_road_curvature_far_distance)  "<i_road_curvature_far_distance>"
  Bus Selector11/7 -> IC/7(R1dC0V)  "<R1dC0V>"
  Bus Selector11/14 -> IC/14(R1bIsLineExis)  "<R1bIsLineExis>"
  Bus Selector11/12 -> IC/12(R1dDisFront)  "<R1dDisFront>"
  Bus Selector11/13 -> IC/13(L1bIsLineExist)  "<L1bIsLineExist>"
  Bus Selector11/3 -> IC/3(L1dC0V)  "<L1dC0V>"
  Bus Selector11/8 -> IC/8(R1dC1V)  "<R1dC1V>"
  Bus Selector11/4 -> IC/4(L1dC1V)  "<L1dC1V>"
  Bus Selector11/19 -> IC/19(i_road_curvature_value_matrix)  "<i_road_curvature_value_matrix>"
  IC/1(accelIC) -> Bus Creator10/1  "accelIC"
  Bus Selector11/10 -> IC/10(R1dC3V)  "<R1dC3V>"
  Bus Selector11/1 -> IC/1(velSubj)  "<velSubj>"
  Bus Selector11/21 -> IC/21(i_road_curvature_matrix_size)  "<i_road_curvature_matrix_size>"
  Bus Selector11/5 -> IC/5(L1dC2V)  "<L1dC2V>"
  Bus Selector11/11 -> IC/11(L1dDisFront)  "<L1dDisFront>"
  IC/5(lowerJerkIC) -> Bus Creator10/5  "lowerJerkIC"
  Bus Selector11/16 -> IC/16(i_road_curvature)  "<i_road_curvature>"
  Bus Selector11/15 -> IC/15(VlcInternalAcc)  "<VlcInternalAccK1>"
  Bus Creator3/1 -> Bus Selector6/1, Bus Selector7/1, Bus Selector10/1, Bus Selector9/1, Bus Selector8/1, Bus Selector5/1, Bus Selector13/1, Bus Selector4/1, Bus Selector11/1
  IC/4(upperJerkIC) -> Bus Creator10/4  "upperJerkIC"
  Bus Selector11/6 -> IC/6(L1dC3V)  "<L1dC3V>"
  Bus Selector11/2 -> IC/2(kap)  "<kap>"
  P_LongCtrltCycle6/1 -> IC/23(tCycle)
  IC/3(lowerBandIC) -> Bus Creator10/3  "lowerBandIC"
  Bus Selector11/20 -> IC/20(i_road_curvature_distance_matrix)  "<i_road_curvature_distance_matrix>"
  Bus Selector11/22 -> IC/22(RFM_UpdateCnt)  "<RFM_UpdateCnt>"
  RFM_UpdateCnt/1 -> Bus Creator3/69  "RFM_UpdateCnt"
  i_road_curvature_matrix_size/1 -> Bus Creator3/52  "i_road_curvature_matrix_size"
  i_road_curvature_far/1 -> Bus Creator3/48  "i_road_curvature_far"
  i_road_curvature_distance_matrix/1 -> Bus Creator3/51  "i_road_curvature_distance_matrix"
  i_road_curvature_value_matrix/1 -> Bus Creator3/50  "i_road_curvature_value_matrix"
  Object_AX/1 -> Bus Creator3/67
  i_road_curvature/1 -> Bus Creator3/47  "i_road_curvature"
  Object_ObstacleProb/1 -> Bus Creator3/65
  i_road_curvature_far_distance/1 -> Bus Creator3/49  "i_road_curvature_far_distance"
  Object_Fus_Type/1 -> Bus Creator3/63
  Object_Type/1 -> Bus Creator3/54
  Object_HeadingAngle/1 -> Bus Creator3/62
  Object_DY/1 -> Bus Creator3/59
  Object_Width/1 -> Bus Creator3/56
  Object_ID/1 -> Bus Creator3/53
  ALC_intention/1 -> Bus Creator3/68  "ALC_intention"
  Object_Length/1 -> Bus Creator3/55
  Object_Age/1 -> Bus Creator3/66
  Object_Hight/1 -> Bus Creator3/57
  Object_DX/1 -> Bus Creator3/58
  Object_VY/1 -> Bus Creator3/61
  Object_VX/1 -> Bus Creator3/60
  Object_ExistProb/1 -> Bus Creator3/64
  Compare To Constant1/1 -> Bus Creator3/23  "SafeStopActive"
  R1dC1V/1 -> Bus Creator3/33  "R1dC1V"
  R1dC0V/1 -> Bus Creator3/32  "R1dC0V"
  L1dC0V/1 -> Bus Creator3/28  "L1dC0V"
  L1dC1V/1 -> Bus Creator3/29  "L1dC1V"
  P3_Exist/1 -> Bus Creator3/44  "P3_Exist"
  L1dDisFront/1 -> Bus Creator3/36  "L1dDisFront"
  R1bIsLineExis/1 -> Bus Creator3/39  "R1bIsLineExis"
  P2_Exist/1 -> Bus Creator3/42  "P2_Exist"
  R1dC3V/1 -> Bus Creator3/35  "R1dC3V"
  R1dDisFront/1 -> Bus Creator3/37  "R1dDisFront"
  distTargRelP3/1 -> Bus Creator3/43  "distTargRelP3"
  velOffRampLimit/1 -> Bus Creator3/45  "velOffRampLimit"
  L1dC3V/1 -> Bus Creator3/31  "L1dC3V"
  L1bIsLineExist/1 -> Bus Creator3/38  "L1bIsLineExist"
  axvRoadSlopeMs2/1 -> Bus Creator3/40  "axvRoadSlopeMs2"
  L1dC2V/1 -> Bus Creator3/30  "L1dC2V"
  distTargRelP2/1 -> Bus Creator3/41  "distTargRelP2"
  distRamp2Cur/1 -> Bus Creator3/46  "distRamp2Cur"
  R1dC2V/1 -> Bus Creator3/34  "R1dC2V"
  FollowCtrl/9(tStartDecel) -> Bus Creator1/9  "tStartDecel"
  Bus Selector7/5 -> FollowCtrl/6(accelTargAbsP0)  "<accelTargAbsP0>"
  Bus Selector6/1 -> VlcInternalAccCalc/1(VlcInternalAccK1)  "<VlcInternalAccK1>"
  Bus Selector8/5 -> SJ/11(velSet)  "<ACC_SpdSetValue>"
  Bus Selector7/2 -> FollowCtrl/3(VlcInternalAccK1)  "<VlcInternalAccK1>"
  Bus Selector8/2 -> SJ/8(TargetExistP0)  "<targetExistP0>"
  Bus Selector8/1 -> SJ/7(velSubj)  "<velSubj>"
  Bus Selector9/1 -> Arbitrate/25(targetExistP0)  "<targetExistP0>"
  Bus Selector8/8 -> SJ/14(timeGapSet)  "<timeGap>"
  Bus Selector10/2 -> AL/7(velSubj)  "<velSubj>"
  Bus Selector10/1 -> AL/6(DrivingMode)  "<LongCtrl_DrivingMode>"
  Bus Selector9/2 -> Arbitrate/26(ACCModeSts)  "<ACCModeSts>"
  IDP2/1 -> Bus Creator3/16  "IDP2"
  accelTargAbsP3/1 -> Bus Creator3/19  "accelTargAbsP3"
  laneChangeEnable/1 -> Bus Creator3/26  "laneChangeEnable"
  P_LongCtrltCycle1/1 -> CCCtrl/11(tCycle)
  Bus Selector12/5 -> Arbitrate/12(lowerJerkIC)  "<lowerJerkIC>"
  IDP3/1 -> Bus Creator3/17  "IDP3"
  SJ/6(ACC_RiTgtObjBarDisp) -> ACC_RiTgtObjBarDisp/1  "ACC_RiTgtObjBarDisp"
  VlcInternalAccK1/1 -> Bus Creator3/7  "VlcInternalAccK1"
  Bus Selector7/1 -> FollowCtrl/2(velSubj)  "<velSubj>"
  Bus Selector4/3 -> CCCtrl/3(IP_VehSpdUnit)  "<IP_VehSpdUnit>"
  P_LongCtrltCycle/1 -> VlcInternalAccCalc/4(tCycle)
  VlcInternalAccCalc/1(VlcInternalAccK20) -> FollowCtrl/1(VlcInternalAccK20)
  Bus Selector6/2 -> VlcInternalAccCalc/2(ACCModeSts)  "<ACCModeSts>"
  Bus Selector15/1 -> tStartDecel/1  "<tStartDecel>"
  Bus Selector3/4 -> SJ/4(distRelDesDistRelPlanNumMin)  "<distRelDesDistRelPlanNumMin>"
  vSetBelowMin/1 -> Bus Creator3/21  "vSetBelowMin"
  Bus Selector4/7 -> CCCtrl/7(SafeStopActive)  "<SafeStopActive>"
  Bus Selector8/9 -> SJ/15(SafeStopActive)  "<SafeStopActive>"
  Bus Selector4/5 -> CCCtrl/5(vSetBelowMin)  "<vSetBelowMin>"
  DrivingMode/1 -> Signal Copy/1
  Arbitrate/3(" lowerBandArb") -> Bus Creator2/3  "lowerBandArb"
  Bus Selector6/3 -> VlcInternalAccCalc/3(accelSubj)  "<accelSubj>"
  Bus Selector/4 -> Arbitrate/4(upperJerkCC)  "<upperJerkCC>"
  Arbitrate/4(" upperJerkArb") -> Bus Creator2/4  "upperJerkArb"
  AL/5(lowerJerkAL) -> lowerJerkAL/1  "lowerJerkAL"
  Bus Selector1/6 -> Arbitrate/23(lowerJerkFollow)  "<lowerJerkFollow>"
  HWAAccControlSts/1 -> Compare To Constant2/1, Compare To Constant1/1, Compare To Constant10/1  "HWAAccControlSts"
  Arbitrate/5(lowerJerkArb) -> Bus Creator2/5  "lowerJerkArb"
  CCCtrl/3(lowerBandCC) -> Bus Creator/3  "lowerBandCC"
  ACC_SpdSetValue/1 -> Bus Creator3/2  "ACC_SpdSetValue"
  FollowCtrl/1(accelFollow) -> Bus Creator1/1  "accelFollow"
  CCCtrl/6(accelCCCtrlAfterJerk) -> Bus Creator/6  "accelCCCtrlAfterJerk"
  Bus Creator/1 -> Bus Selector/1
  Bus Creator5/1 -> Bus Selector14/1
  Bus Selector7/8 -> FollowCtrl/9(IDP0)  "<IDP0>"
  Bus Selector8/6 -> SJ/12(ACCModeSts)  "<ACCModeSts>"
  ORD/1(accelORD) -> Bus Creator5/1  "accelORD"
  FollowCtrl/2(upperBandFollow) -> Bus Creator1/2  "upperBandFollow"
  AL/1(accelAL) -> accelAL/1  "accelAL"
  Bus Selector/3 -> Arbitrate/3(lowerBandCC)  "<lowerBandCC>"
  ORD/3(lowerBandORD) -> Bus Creator5/3  "lowerBandORD"
  ORD/2(upperBandORD) -> Bus Creator5/2  "upperBandORD"
  Bus Selector7/7 -> FollowCtrl/8(ACCModeSts)  "<ACCModeSts>"
  SJ/7(DriveOffConditonFulfilled) -> [DriveOffConditonFulfilled], DriveOffConditonFulfilled/1  "DriveOffConditonFulfilled"
  velSubj/1 -> Bus Creator3/8  "velSubj"
  Arbitrate/1(accelArb) -> Bus Creator2/1  "accelArb"
  Bus Selector13/1 -> ORD/1(velOffRampLimit)  "<velOffRampLimit>"
  SJ/3(tor) -> tor/1  "tor"
  Arbitrate/2(" upperBandArb") -> Bus Creator2/2  "upperBandArb"
  Bus Selector4/2 -> CCCtrl/2(VehicleSpd)  "<vehicleSpd>"
  Bus Selector/5 -> Arbitrate/5(lowerJerkCC)  "<lowerJerkCC>"
  Bus Selector/2 -> Arbitrate/2(upperBandCC)  "<upperBandCC>"
  Bus Selector7/3 -> FollowCtrl/4(distTargRel)  "<distTargRel>"
  Bus Selector5/1 -> TargetUpdate/1(TOS_UpdateCnt)  "<TOS_UpdateCnt>"
  Bus Selector8/12 -> SJ/18(distTargRelP3)  "<distTargRelP3>"
  CCCtrl/2(upperBandCC) -> Bus Creator/2  "upperBandCC"
  Unit Delay/1 -> FollowCtrl/19(DrvOFF_Req)
  Bus Selector2/1 -> AL/1(accelArb)  "<accelArb>"
  Bus Selector7/4 -> FollowCtrl/5(velTargRel)  "<velTargRel>"
  ORD/5(lowerJerkORD) -> Bus Creator5/5  "lowerJerkORD"
  Bus Selector7/15 -> FollowCtrl/16(axvRoadSlopeMs2)  "<axvRoadSlopeMs2>"
  FollowCtrl/7(distRelDesDistRelPlanNumMin) -> Bus Creator1/7  "distRelDesDistRelPlanNumMin"
  Bus Selector13/2 -> ORD/2(distRamp2Cur)  "<distRamp2Cur>"
  Bus Selector14/4 -> Arbitrate/16(upperJerkORD)  "<upperJerkORD>"
  Bus Selector14/5 -> Arbitrate/17(lowerJerkORD)  "<lowerJerkORD>"
  Bus Selector4/1 -> CCCtrl/1(ACC_SpdSetValue)  "<ACC_SpdSetValue>"
  CCCtrl/4(upperJerkCC) -> Bus Creator/4  "upperJerkCC"
  ORD/4(upperJerkORD) -> Bus Creator5/4  "upperJerkORD"
  Bus Selector7/14 -> FollowCtrl/15(laneChangeEnable)  "<laneChangeEnable>"
  SJ/5(ACC_LeTgtObjBarDisp) -> ACC_LeTgtObjBarDisp/1  "ACC_LeTgtObjBarDisp"
  Bus Selector14/2 -> Arbitrate/14(upperBandORD)  "<upperBandORD>"
  Bus Selector14/3 -> Arbitrate/15(lowerBandORD)  "<lowerBandORD>"
  Bus Creator10/1 -> Bus Selector12/1
  Bus Selector13/3 -> ORD/3(vehicleSpd)  "<vehicleSpd>"
  dangerLevel/1 -> Bus Creator3/25  "dangerLevel"
  Bus Selector12/2 -> Arbitrate/9(upperBandIC)  "<upperBandIC>"
  Constant/1 -> Bus Creator3/5  "IP_VehSpdUnit"
  Bus Selector/6 -> Arbitrate/6(accelCCCtrlAfterJerk)  "<accelCCCtrlAfterJerk>"
  Bus Selector7/6 -> FollowCtrl/7(timeGap)  "<timeGap>"
  Bus Selector7/13 -> FollowCtrl/14(dangerLevel)  "<dangerLevel>"
  Bus Selector4/4 -> CCCtrl/4(VlcInternalAccK1)  "<VlcInternalAccK1>"
  FollowCtrl/5(lowerJerkFollow) -> Bus Creator1/5  "lowerJerkFollow"
  FollowtCycle/1 -> FollowCtrl/18(tCycle)
  accelSubj/1 -> Bus Creator3/9  "accelSubj"
  Bus Selector8/7 -> SJ/13(VlcInternalAcc)  "<VlcInternalAccK1>"
  timeGap/1 -> Bus Creator3/13  "timeGap"
  SJ/4(ACC_TgtObjBarDisp) -> ACC_TgtObjBarDisp/1  "ACC_TgtObjBarDisp"
  TOS_UpdateCnt/1 -> Bus Creator3/15  "TOS_UpdateCnt"
  Compare To Constant10/1 -> Bus Creator3/22  "HWAIsLaneChange"
  Bus Selector3/3 -> SJ/3(distRelPlanMin)  "<distRelPlanMin>"
  Bus Selector14/1 -> Arbitrate/13(accelORD)  "<accelORD>"
  Bus Selector4/6 -> CCCtrl/6(IsLaneChange)  "<HWAIsLaneChange>"
  IDP0/1 -> Bus Creator3/14  "IDP0"
  Bus Selector1/3 -> Arbitrate/20(upperBandFollow)  "<upperBandFollow>"
  accelTargAbsP2/1 -> Bus Creator3/18  "accelTargAbsP2"
  accelTargAbsP0/1 -> Bus Creator3/12  "accelTargAbsP0"
  Bus Selector1/4 -> Arbitrate/21(lowerBandFollow)  "<lowerBandFollow>"
  kap/1 -> Bus Creator3/27  "kap"
  distTargRel/1 -> Bus Creator3/10  "distTargRel"
  Bus Selector8/4 -> SJ/10(velTargetRel)  "<velTargRel>"
  Bus Selector1/2 -> Arbitrate/19(accelFollowAfterJerk)  "<accelFollowAfterJerk>"
  FollowCtrl/10(accelFollowAfterJerk) -> Bus Creator1/10  "accelFollowAfterJerk"
  Bus Creator1/1 -> Bus Selector3/1, Bus Selector15/1, Bus Selector1/1
  VehicleSpd/1 -> Bus Creator3/4  "vehicleSpd"
  FollowCtrl/4(upperJerkFollow) -> Bus Creator1/4  "upperJerkFollow"
  targetExistP0/1 -> Bus Creator3/1  "targetExistP0"
  [DriveOffConditonFulfilled] -> Unit Delay/1
  Bus Selector8/3 -> SJ/9(distTargRel)  "<distTargRel>"
  AL/4(upperJerkAL) -> upperJerkAL/1  "upperJerkAL"
  SJ/2(BrakePrefer) -> BrakePrefer/1  "BrakePrefer"
  Bus Selector12/4 -> Arbitrate/11(upperJerkIC)  "<upperJerkIC>"
  Bus Selector2/4 -> AL/4(upperJerkArb)  "<upperJerkArb>"
  Subsystem/1(ACCModeSts) -> Bus Creator3/3  "ACCModeSts"
  Bus Selector8/11 -> SJ/17(P2_Exist)  "<P2_Exist>"
  Bus Selector8/10 -> SJ/16(distTargRelP2)  "<distTargRelP2>"
  FollowCtrl/6(distRelPlanMin) -> Bus Creator1/6  "distRelPlanMin"
  Bus Selector12/1 -> Arbitrate/8(accelIC)  "<accelIC>"
  Bus Selector2/5 -> AL/5(lowerJerkArb)  "<lowerJerkArb>"
  Bus Selector3/2 -> SJ/2(distDesCur)  "<distDesCur>"
  CCCtrl/1(accelCC) -> Bus Creator/1  "accelCC"
  CCCtrl/5(lowerJerkCC) -> Bus Creator/5  "lowerJerkCC"
  SJ/1(DecleToStop) -> DecleToStop/1  "DecleToStop"
  velTargRel/1 -> Bus Creator3/11  "velTargRel"
  Bus Selector/1 -> Arbitrate/1(accelCC)  "<accelCC>"
  Bus Selector7/9 -> FollowCtrl/10(IDP2)  "<IDP2>"
  Bus Selector3/1 -> SJ/1(accelFollow)  "<accelFollow>"
  Bus Selector8/13 -> SJ/19(P3_Exist)  "<P3_Exist>"
  TargetUpdate/1(targUpdate) -> FollowCtrl/Enable
  FollowCtrl/3(lowerBandFollow) -> Bus Creator1/3  "lowerBandFollow"
  Bus Selector1/5 -> Arbitrate/22(upperJerkFollow)  "<upperJerkFollow>"
  Bus Selector7/10 -> FollowCtrl/11(IDP3)  "<IDP3>"
  AL/2(upperBandAL) -> upperBandAL/1  "upperBandAL"
  Bus Selector2/3 -> AL/3(lowerBandArb)  "<lowerBandArb>"
  Bus Creator2/1 -> Bus Selector2/1
  Bus Selector1/1 -> Arbitrate/18(accelFollow)  "<accelFollow>"
  Bus Selector7/11 -> FollowCtrl/12(accelTargAbsP2)  "<accelTargAbsP2>"
  Bus Selector2/2 -> AL/2(upperBandArb)  "<upperBandArb>"
  AL/3(lowerBandAL) -> lowerBandAL/1  "lowerBandAL"
  Bus Selector12/3 -> Arbitrate/10(lowerBandIC)  "<lowerBandIC>"
  FollowCtrl/8(distDesCur) -> Bus Creator1/8  "distDesCur"
  Bus Selector7/12 -> FollowCtrl/13(accelTargAbsP3)  "<accelTargAbsP3>"
  Bus Selector8/14 -> SJ/20(axvRoadSlopeMs2)  "<axvRoadSlopeMs2>"
  Bus Selector4/8 -> CCCtrl/8(DrivingMode)  "<LongCtrl_DrivingMode>"
  Bus Selector4/9 -> CCCtrl/9(velSubj)  "<velSubj>"
  CCCtrl/7(velSubjPlanCC2ALC) -> Bus Creator/7  "velSubjPlanCC2ALC"
  Arbitrate/6(velPlanEffect) -> velPlanEffect/1  "velPlanEffect"
  FollowCtrl/11(velSubjPlanFollow) -> Bus Creator1/11  "velSubjPlanFollow"
  Bus Selector/7 -> Arbitrate/7(velSubjPlanCC)  "<velSubjPlanCC2ALC>"
  Bus Selector1/7 -> Arbitrate/24(velSubjPlanFollow)  "<velSubjPlanFollow>"
  Arbitrate/7(velSubjPlanArb) -> velSubjPlanArb/1
  FollowCtrl/12(ttc) -> Bus Creator1/12  "ttc"
  FollowCtrl/13(accelSubjPlanOpt) -> Bus Creator1/13  "accelSubjPlanOpt"
  Bus Selector3/5 -> SJ/5(ttc)  "<ttc>"
  Bus Selector3/6 -> SJ/6(accelSubjPlanOpt)  "<accelSubjPlanOpt>"
  Bus Selector8/15 -> SJ/21(accelSubj)  "<accelSubj>"
  Bus Selector8/16 -> SJ/22(VlcInternalAccK1)  "<VlcInternalAccK1>"
  Compare To Constant2/1 -> Bus Creator3/24  "HWASlowQuit"
  Bus Selector8/17 -> SJ/23(HWASlowQuit)  "<HWASlowQuit>"
  laneChangeIncSetSpdReq/1 -> Bus Creator3/70  "laneChangeIncSetSpdReq"
  Bus Selector4/10 -> CCCtrl/10(laneChangeIncSetSpdReq)  "<laneChangeIncSetSpdReq>"

== system PvtSubSys_PLAN_AP/AP/AP/AL ==
  accelArb : Inport
  upperBandArb : Inport  Port=2
  lowerBandArb : Inport  Port=3
  upperJerkArb : Inport  Port=4
  lowerJerkArb : Inport  Port=5
  DrivingMode : Inport  Port=6
  velSubj : Inport  Port=7  OutDataTypeStr=single
  HWASlowQuit : Inport  Port=8
  AL : Stateflow chart  TreatAsAtomicUnit=on
  AcceLowerLimitChar : simulink/Lookup Tables/Lookup Table Dynamic  LookUpMeth=Interpolation-Use End Values  OutDataType=fixdt('single')  OutScaling=[]  OutputDataTypeScalingMode=Specify via dialog  OutDataTypeStr=single  DoSatur=off
  AcceUpperLimitEcoModeChar : simulink/Lookup Tables/Lookup Table Dynamic  LookUpMeth=Interpolation-Use End Values  OutDataType=fixdt('single')  OutScaling=[]  OutputDataTypeScalingMode=Specify via dialog  OutDataTypeStr=single  DoSatur=off
  AcceUpperLimitNormalModeChar : simulink/Lookup Tables/Lookup Table Dynamic  LookUpMeth=Interpolation-Use End Values  OutDataType=fixdt('single')  OutScaling=[]  OutputDataTypeScalingMode=Specify via dialog  OutDataTypeStr=single  DoSatur=off
  AcceUpperLimitSportModeChar : simulink/Lookup Tables/Lookup Table Dynamic  LookUpMeth=Interpolation-Use End Values  OutDataType=fixdt('single')  OutScaling=[]  OutputDataTypeScalingMode=Specify via dialog  OutDataTypeStr=single  DoSatur=off
  Bus Creator : BusCreator  Inputs=4
  Bus Selector : BusSelector  OutputSignals=AcceUpperLimitNormalMode,AcceUpperLimitSportMode,AcceUpperLimitEcoMode,AcceLowerLimit
  PALaLowerChar : Constant  Value=P_LongCtrl_ALaLowerChar
  P_LongCtrl_ALaUpperCharEco : Constant  Value=P_LongCtrl_ALaUpperCharEco
  P_LongCtrl_ALaUpperCharNormal : Constant  Value=P_LongCtrl_ALaUpperCharNormal
  P_LongCtrl_ALaUpperCharSport : Constant  Value=P_LongCtrl_ALaUpperCharSport
  P_LongCtrl_ALvAcceleLowerChar : Constant  Value=P_LongCtrl_ALvAcceleLowerChar
  P_LongCtrl_ALvAcceleUpperCharEco : Constant  Value=P_LongCtrl_ALvAcceleUpperCharEco
  P_LongCtrl_ALvAcceleUpperCharNormal : Constant  Value=P_LongCtrl_ALvAcceleUpperCharNormal
  P_LongCtrl_ALvAcceleUpperCharSport : Constant  Value=P_LongCtrl_ALvAcceleUpperCharSport
  accelAL : Outport  OutDataTypeStr=single
  upperBandAL : Outport  Port=2  OutDataTypeStr=single
  lowerBandAL : Outport  Port=3  OutDataTypeStr=single
  upperJerkAL : Outport  Port=4  OutDataTypeStr=single
  lowerJerkAL : Outport  Port=5  OutDataTypeStr=single
  wires:
  HWASlowQuit/1 -> AL/11(HWASlowQuit)  "HWASlowQuit"
  AL/5(lowerJerkAL) -> lowerJerkAL/1  "LongCtrl_lowerJerkAL"
  AL/4(upperJerkAL) -> upperJerkAL/1  "LongCtrl_upperJerkAL"
  AL/3(lowerBandAL) -> lowerBandAL/1  "LongCtrl_lowerBandAL"
  AL/2(upperBandAL) -> upperBandAL/1  "LongCtrl_upperBandAL"
  AL/1(accelAL) -> accelAL/1  "LongCtrl_accelAL"
  lowerJerkArb/1 -> AL/10(lowerJerkArb)  "lowerJerkArb"
  upperJerkArb/1 -> AL/9(upperJerkArb)  "upperJerkArb"
  lowerBandArb/1 -> AL/8(lowerBandArb)  "lowerBandArb"
  upperBandArb/1 -> AL/7(upperBandArb)  "upperBandArb"
  accelArb/1 -> AL/6(accelArb)  "accelArb"
  DrivingMode/1 -> AL/5(DrivingMode)  "DrivingMode"
  Bus Selector/4 -> AL/4(AcceLowerLimit)  "<AcceLowerLimit>"
  Bus Selector/3 -> AL/3(AcceUpperLimitEcoMode)  "<AcceUpperLimitEcoMode>"
  Bus Selector/1 -> AL/1(AcceUpperLimitNormalMode)  "<AcceUpperLimitNormalMode>"
  Bus Selector/2 -> AL/2(AcceUpperLimitSportMode)  "<AcceUpperLimitSportMode>"
  Bus Creator/1 -> Bus Selector/1
  AcceUpperLimitNormalModeChar/1 -> Bus Creator/1  "AcceUpperLimitNormalMode"
  AcceUpperLimitSportModeChar/1 -> Bus Creator/2  "AcceUpperLimitSportMode"
  AcceLowerLimitChar/1 -> Bus Creator/4  "AcceLowerLimit"
  AcceUpperLimitEcoModeChar/1 -> Bus Creator/3  "AcceUpperLimitEcoMode"
  velSubj/1 -> AcceUpperLimitNormalModeChar/1, AcceUpperLimitSportModeChar/1, AcceUpperLimitEcoModeChar/1, AcceLowerLimitChar/1  "velSubj"
  P_LongCtrl_ALvAcceleLowerChar/1 -> AcceLowerLimitChar/2
  PALaLowerChar/1 -> AcceLowerLimitChar/3
  P_LongCtrl_ALaUpperCharEco/1 -> AcceUpperLimitEcoModeChar/3
  P_LongCtrl_ALvAcceleUpperCharEco/1 -> AcceUpperLimitEcoModeChar/2
  P_LongCtrl_ALvAcceleUpperCharSport/1 -> AcceUpperLimitSportModeChar/2
  P_LongCtrl_ALaUpperCharSport/1 -> AcceUpperLimitSportModeChar/3
  P_LongCtrl_ALaUpperCharNormal/1 -> AcceUpperLimitNormalModeChar/3
  P_LongCtrl_ALvAcceleUpperCharNormal/1 -> AcceUpperLimitNormalModeChar/2
